simulink model "DESHAN_2022E039"  (R2024a)
settings: Solver=VariableStepAuto  StartTime=0.0  StopTime=10.0  RelTol=1e-3
libraries: dspfdesign x1
settings Model: Creator=dcrea  LastModifiedBy=dcrea

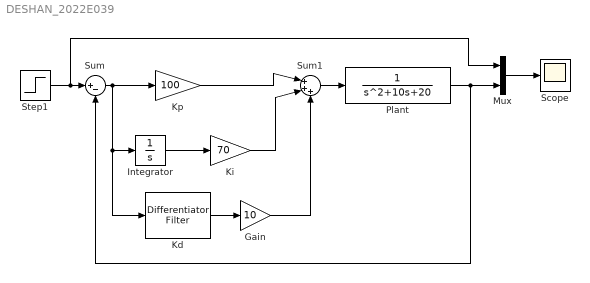
== system DESHAN_2022E039 ==
  " Scope" : Scope
  Gain : Gain  Gain=10
  Integrator : Integrator
  Kd : dspfdesign/Differentiator Filter  DesignForMinimumOrder=on  FilterOrder=31  PassbandRipple=0.1  ScaleCoefficients=off  SimulateUsing=Interpreted execution  roundingMode=Floor  coeffsDataTypeStr=fixdt(1,16)
  Ki : Gain  Gain=70
  Kp : Gain  Gain=100
  Mux : Mux  Inputs=2
  Plant : TransferFcn  Denominator=[1 10 20]
  Step1 : Step  SampleTime=0
  Sum : Sum  Inputs=|+-
  Sum1 : Sum  Inputs=|+++
  wires:
  Sum/1 -> Kd/1, Integrator/1, Kp/1
  Plant/1 -> Mux/2, Sum/2
  Integrator/1 -> Ki/1
  Kp/1 -> Sum1/1
  Sum1/1 -> Plant/1
  Kd/1 -> Gain/1
  Gain/1 -> Sum1/3
  Ki/1 -> Sum1/2
  Step1/1 -> Mux/1, Sum/1
  Mux/1 -> " Scope"/1
